simulink model "helimodel_mpc"  (Simulink 6.2)
settings: Solver=ode45  StartTime=0.0  StopTime=50  RelTol=1e-3
values from neighbouring files (symbols this model uses):
  elev_max = 0.6    [Simulate_Helicopter_MPC.m]
  elev_min = -0.5    [Simulate_Helicopter_MPC.m]
  Fg = 0.5    [Simulate_Helicopter_MPC.m]
  Je = 0.91    [Simulate_Helicopter_MPC.m]
  Jp = 0.0364    [Simulate_Helicopter_MPC.m]
  Jt = Je    (= 0.91)    [Simulate_Helicopter_MPC.m]
  Kf = 0.5    [Simulate_Helicopter_MPC.m]
  la = 0.66    [Simulate_Helicopter_MPC.m]
  lh = 0.177    [Simulate_Helicopter_MPC.m]
  md = MPCInit(Ad,Bd,Cd,Cz,Dz,Cc,Dc,Hp,Hw,z_blk,Hu,u_blk, 	     du_max,du_min,u_max,u_min,z_max,z_min,Q,R,[],[],h,cmode,  	     'qp_ip')    [Simulate_Helicopter_MPC.m]
  pitch_max = 1    [Simulate_Helicopter_MPC.m]
  pitch_min = -1    [Simulate_Helicopter_MPC.m]
  Tg = la*Fg    (= 0.33)    [Simulate_Helicopter_MPC.m]
  u1_max = 3    [Simulate_Helicopter_MPC.m]
  u1_min = -2    [Simulate_Helicopter_MPC.m]
  u2_max = 3    [Simulate_Helicopter_MPC.m]
  u2_min = -2    [Simulate_Helicopter_MPC.m]
  u_stat = [Tg/(2*Kf*la) Tg/(2*Kf*la)]'    [Simulate_Helicopter_MPC.m]
  x0 = x_stat    [Simulate_Helicopter_MPC.m]
  x_stat = [0 0 0 0 0 0]'    [Simulate_Helicopter_MPC.m]
settings Model: Creator=jakesson  LastModifiedBy=jakesson  ExtModeAutoUpdateStatusClock=off
settings DataIOCC: SignalLoggingName=sigsOut  Refine=10
settings HardwareCC: TargetUnknown=on

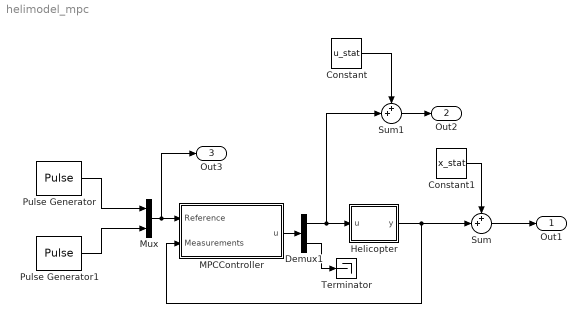
== system helimodel_mpc ==
  Constant : Constant  Value=u_stat
  Constant1 : Constant  Value=x_stat
  Demux1 : Demux  Outputs=[2 6]
  Helicopter : Subsystem
  MPCController : Subsystem  mask{md=md}
      mask prompts: md "MPCData"
  Mux : Mux  Inputs=2
  Pulse Generator : DiscretePulseGenerator  PulseType=Time based  Amplitude=0.3  Period=15  PulseWidth=50
  Pulse Generator1 : DiscretePulseGenerator  PulseType=Time based  Amplitude=3  Period=30  PulseWidth=50
  Sum : Sum  Inputs=++|  SaturateOnIntegerOverflow=on
  Sum1 : Sum  Inputs=++|  SaturateOnIntegerOverflow=on
  Terminator : Terminator
  Out1 : Outport
  Out2 : Outport  Port=2
  Out3 : Outport  Port=3
  wires:
  MPCController/1(u) -> Demux1/1
  Mux/1 -> MPCController/1(Reference), Out3/1
  Helicopter/1(y) -> MPCController/2(Measurements), Sum/2
  Pulse Generator/1 -> Mux/1
  Pulse Generator1/1 -> Mux/2
  Demux1/1 -> Helicopter/1(u), Sum1/2
  Demux1/2 -> Terminator/1
  Constant1/1 -> Sum/1
  Sum/1 -> Out1/1
  Constant/1 -> Sum1/1
  Sum1/1 -> Out2/1

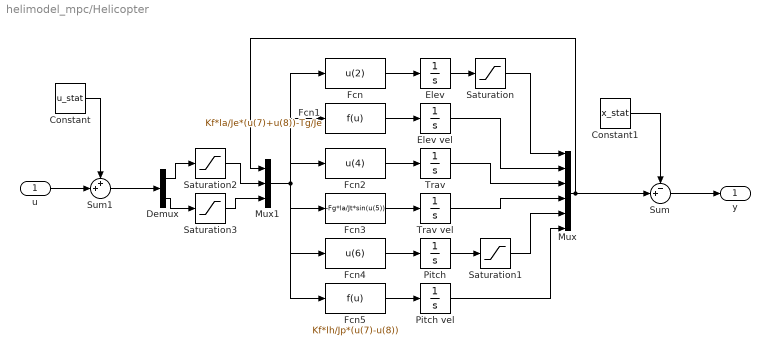
== system helimodel_mpc/Helicopter ==
  u : Inport  Port=1  LatchInput=off
  Constant : Constant  Value=u_stat
  Constant1 : Constant  Value=x_stat
  Demux : Demux  Outputs=2
  Elev : Integrator  InitialCondition=x0(1)
  Elev vel : Integrator  InitialCondition=x0(2)
  Fcn : Fcn  Expr=u(2)
  Fcn1 : Fcn  Expr=Kf*la/Je*(u(7)+u(8))-Tg/Je
  Fcn2 : Fcn  Expr=u(4)
  Fcn3 : Fcn  Expr=-Fg*la/Jt*sin(u(5))
  Fcn4 : Fcn  Expr=u(6)
  Fcn5 : Fcn  Expr=Kf*lh/Jp*(u(7)-u(8))
  Mux : Mux  Inputs=6
  Mux1 : Mux  Inputs=3
  Pitch : Integrator  InitialCondition=x0(5)
  Pitch vel : Integrator  InitialCondition=x0(6)
  Saturation : Saturate  UpperLimit=elev_max  LowerLimit=elev_min
  Saturation1 : Saturate  UpperLimit=pitch_max  LowerLimit=pitch_min
  Saturation2 : Saturate  UpperLimit=u1_max  LowerLimit=u1_min
  Saturation3 : Saturate  UpperLimit=u2_max  LowerLimit=u2_min
  Sum : Sum  Inputs=-+|  SaturateOnIntegerOverflow=on
  Sum1 : Sum  Inputs=++|  SaturateOnIntegerOverflow=on
  Trav : Integrator  InitialCondition=x0(3)
  Trav vel : Integrator  InitialCondition=x0(4)
  y : Outport
  wires:
  Saturation3/1 -> Mux1/3
  Saturation2/1 -> Mux1/2
  Demux/2 -> Saturation3/1
  Demux/1 -> Saturation2/1
  Mux/1 -> Mux1/1, Sum/2
  Mux1/1 -> Fcn5/1, Fcn4/1, Fcn2/1, Fcn3/1, Fcn1/1, Fcn/1
  Fcn5/1 -> Pitch vel/1
  Fcn4/1 -> Pitch/1
  Fcn3/1 -> Trav vel/1
  Fcn2/1 -> Trav/1
  Fcn1/1 -> Elev vel/1
  Fcn/1 -> Elev/1
  Pitch vel/1 -> Mux/6
  Saturation1/1 -> Mux/5
  Trav vel/1 -> Mux/4
  Trav/1 -> Mux/3
  Elev vel/1 -> Mux/2
  Saturation/1 -> Mux/1
  Elev/1 -> Saturation/1
  Pitch/1 -> Saturation1/1
  Sum1/1 -> Demux/1
  u/1 -> Sum1/2
  Constant/1 -> Sum1/1
  Constant1/1 -> Sum/1
  Sum/1 -> y/1

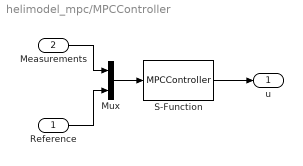
== system helimodel_mpc/MPCController ==
  Reference : Inport  Port=1  LatchInput=off
  Measurements : Inport  Port=2  LatchInput=off
  Mux : Mux  Inputs=2
  S-Function : S-Function  FunctionName=MPCController  Parameters=md
  u : Outport
  wires:
  S-Function/1 -> u/1
  Reference/1 -> Mux/2
  Measurements/1 -> Mux/1
  Mux/1 -> S-Function/1
